simulink model "EV_ControlSystem_Architecture"  (R2025b)
settings: Solver=FixedStepAuto  StartTime=0.0  StopTime=inf  RelTol=1e-3
settings Model: DataDictionary=systemParams.sldd  Creator=smuckati  LastModifiedBy=smuckati
settings OptimizationCC: UseDivisionForNetSlopeComputation=on
settings DebuggingCC: ParameterPrecisionLossMsg=none
settings ModelReferenceCC: ModelReferenceNumInstancesAllowed=Single
settings RTWCC: GPUComputeCapability=3.5
settings GRTTargetCC: SubcomponentCodeInterfacePackaging=Nonreusable function

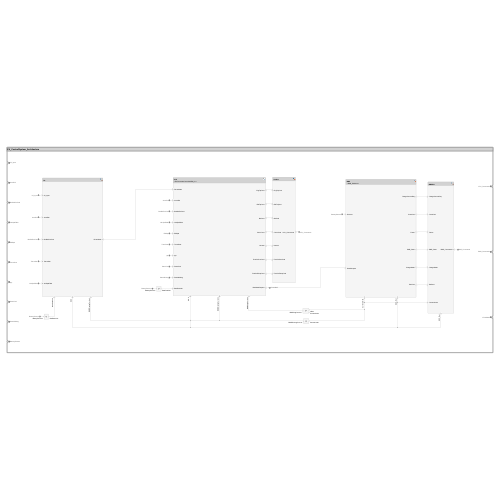
[thumbnail: Simulink's stored preview of the top-level diagram]
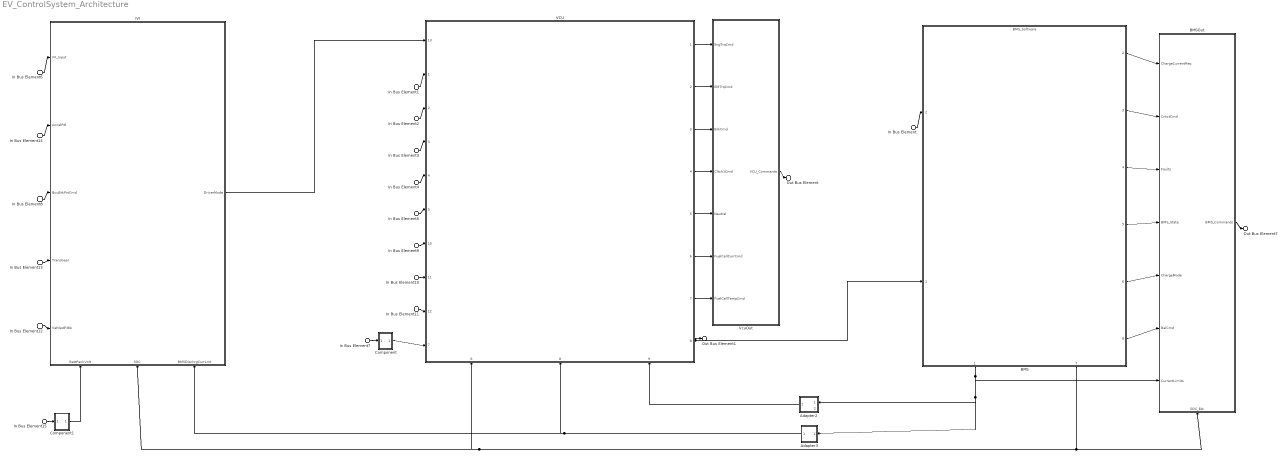
== system EV_ControlSystem_Architecture ==
  In Bus Element6 : Inport  PortName=IVI_Input
  In Bus Element1 : Inport  Port=2  PortName=AccelPdl
  In Bus Element14 : Inport  Port=2  PortName=AccelPdl
  In Bus Element2 : Inport  Port=3  PortName=BcuBrkPrsCmd
  In Bus Element8 : Inport  Port=3  PortName=BcuBrkPrsCmd
  In Bus Element3 : Inport  Port=4  PortName=VehSpdFdbk
  In Bus Element12 : Inport  Port=4  PortName=VehSpdFdbk
  In Bus Element4 : Inport  Port=5  PortName=EMSpd
  In Bus Element5 : Inport  Port=6  PortName=TransGear
  In Bus Element13 : Inport  Port=6  PortName=TransGear
  In Bus Element9 : Inport  Port=7  PortName=pqr
  In Bus Element10 : Inport  Port=8  PortName=SteerCmd
  In Bus Element11 : Inport  Port=9  PortName=SteerWhlAng
  In Bus Element : Inport  Port=10  PortName=BatterySensors
  In Bus Element7 : Inport  Port=10  PortName=BatterySensors
  In Bus Element15 : Inport  Port=10  PortName=BatterySensors
  Adapter2 : Subsystem
      settings: PortSchema="{\"entries\":[{\"content\":{\"margin\":10,\"minimumSpacing\":15,\"sides\":[{\"content\":{\"connectorIds\":[\"Out1\"]},\"type\":\"ConnectorPlacement.EquallySpacedRectSide\",\"uuid\":\"0bbc9e3d-7235-47d6-ad6f-dd1f8eb5ef8f\"},{\"content\":{\"connectorIds\":[\"In1\",\"In2\"],\"side\":\"RIGHT\"},\"type\":\"ConnectorPlacement.EquallySpacedRectSide\",\"uuid\":\"65cf6885-6ff6-4737-9f0f-48431dc9ec05\"},{\"content\":{\"side\":\"TOP\"},\"type\":\"ConnectorPlacement.EquallySpacedRectSide\",\"uuid\":\"345e4547-f67c-4bab-8588-ce41d45f9363\"}]},\"type\":\"ConnectorPlacement.EquallySpacedConnector\",\"uuid\":\"b8001fcd-770d-4504-9144-d19717d53d24\"}],\"packageUris\":[\"http://schema.mathworks.com/mf0/Connector/R2020b\"],\"version\":\"1.0\"}"
  Adapter3 : Subsystem
      settings: PortSchema="{\"entries\":[{\"content\":{\"margin\":10,\"minimumSpacing\":15,\"sides\":[{\"content\":{\"connectorIds\":[\"Out1\"]},\"type\":\"ConnectorPlacement.EquallySpacedRectSide\",\"uuid\":\"0bbc9e3d-7235-47d6-ad6f-dd1f8eb5ef8f\"},{\"content\":{\"connectorIds\":[\"In1\"],\"side\":\"RIGHT\"},\"type\":\"ConnectorPlacement.EquallySpacedRectSide\",\"uuid\":\"65cf6885-6ff6-4737-9f0f-48431dc9ec05\"},{\"content\":{\"side\":\"TOP\"},\"type\":\"ConnectorPlacement.EquallySpacedRectSide\",\"uuid\":\"345e4547-f67c-4bab-8588-ce41d45f9363\"}]},\"type\":\"ConnectorPlacement.EquallySpacedConnector\",\"uuid\":\"b8001fcd-770d-4504-9144-d19717d53d24\"}],\"packageUris\":[\"http://schema.mathworks.com/mf0/Connector/R2020b\"],\"version\":\"1.0\"}"
  BMS : ModelReference  ModelNameDialog=BMS_Software  SimulationMode=Normal  ModelReferenceVersion=11.4
      settings: PortSchema="{\"entries\":[{\"content\":{\"headerSize\":38,\"margin\":15,\"minimumSpacing\":25,\"sides\":[{\"content\":{\"connectorIds\":[\"In2\",\"In1\"]},\"type\":\"ConnectorPlacement.EquallySpacedRectSide\",\"uuid\":\"1684aa06-7c09-45e9-a207-933b45b16ad6\"},{\"content\":{\"connectorIds\":[\"Out2\",\"Out3\",\"Out4\",\"Out5\",\"Out6\",\"Out8\"],\"side\":\"RIGHT\"},\"type\":\"ConnectorPlacement.EquallySpacedRectSide\",\"uuid\":\"92a40eb6-ce6d-4197-95e5-619e5cbf745b\"},{\"content\":{\"side\":\"TOP\"},\"type\":\"ConnectorPlacement.EquallySpacedRectSide\",\"uuid\":\"e9ffeedd-dc68-477a-803d-14826416b02e\"},{\"content\":{\"connectorIds\":[\"Out1\",\"Out7\"],\"side\":\"BOTTOM\"},\"type\":\"ConnectorPlacement.EquallySpacedRectSide\",\"uuid\":\"a73cbf5d-dd2f-4f3b-b4a2-8c33c0d9382e\"}]},\"type\":\"ConnectorPlacement.EquallySpacedConnector\",\"uuid\":\"1901e345-f71e-4164-ad80-cf1092e39a7b\"}],\"packageUris\":[\"http://schema.mathworks.com/mf0/Connector/R2020b\"],\"version\":\"1.0\"}"
  BMSOut : Subsystem
      settings: PortSchema="{\"entries\":[{\"content\":{\"headerSize\":26,\"margin\":15,\"minimumSpacing\":25,\"sides\":[{\"content\":{\"connectorIds\":[\"In2\",\"In3\",\"In4\",\"In5\",\"In6\",\"In7\",\"In8\"]},\"type\":\"ConnectorPlacement.EquallySpacedRectSide\",\"uuid\":\"58a5bcb5-b5b6-43c9-9ab9-ad7b56807429\"},{\"content\":{\"connectorIds\":[\"Out1\"],\"side\":\"RIGHT\"},\"type\":\"ConnectorPlacement.EquallySpacedRectSide\",\"uuid\":\"182e3572-20a9-4903-88bd-08ae5ae4a66b\"},{\"content\":{\"side\":\"TOP\"},\"type\":\"ConnectorPlacement.EquallySpacedRectSide\",\"uuid\":\"b57b91fb-4a21-4ebf-b0d2-47c47f92b1a1\"},{\"content\":{\"connectorIds\":[\"In1\"],\"side\":\"BOTTOM\"},\"type\":\"ConnectorPlacement.EquallySpacedRectSide\",\"uuid\":\"ffc923e8-341b-44c7-96b0-eae8ed13ab76\"}]},\"type\":\"ConnectorPlacement.EquallySpacedConnector\",\"uuid\":\"fd34c378-6982-409c-b390-5cad93b9488e\"}],\"packageUris\":[\"http://schema.mathworks.com/mf0/Connector/R2020b\"],\"version\":\"1.0\"}"
  Component : Subsystem
      settings: PortSchema="{\"entries\":[{\"content\":{\"margin\":10,\"minimumSpacing\":15,\"sides\":[{\"content\":{\"connectorIds\":[\"In1\"]},\"type\":\"ConnectorPlacement.EquallySpacedRectSide\",\"uuid\":\"0bbc9e3d-7235-47d6-ad6f-dd1f8eb5ef8f\"},{\"content\":{\"connectorIds\":[\"Out1\"],\"side\":\"RIGHT\"},\"type\":\"ConnectorPlacement.EquallySpacedRectSide\",\"uuid\":\"65cf6885-6ff6-4737-9f0f-48431dc9ec05\"},{\"content\":{\"side\":\"TOP\"},\"type\":\"ConnectorPlacement.EquallySpacedRectSide\",\"uuid\":\"345e4547-f67c-4bab-8588-ce41d45f9363\"}]},\"type\":\"ConnectorPlacement.EquallySpacedConnector\",\"uuid\":\"b8001fcd-770d-4504-9144-d19717d53d24\"}],\"packageUris\":[\"http://schema.mathworks.com/mf0/Connector/R2020b\"],\"version\":\"1.0\"}"
  Component1 : Subsystem
      settings: PortSchema="{\"entries\":[{\"content\":{\"margin\":10,\"minimumSpacing\":15,\"sides\":[{\"content\":{\"connectorIds\":[\"In1\"]},\"type\":\"ConnectorPlacement.EquallySpacedRectSide\",\"uuid\":\"0bbc9e3d-7235-47d6-ad6f-dd1f8eb5ef8f\"},{\"content\":{\"connectorIds\":[\"Out1\"],\"side\":\"RIGHT\"},\"type\":\"ConnectorPlacement.EquallySpacedRectSide\",\"uuid\":\"65cf6885-6ff6-4737-9f0f-48431dc9ec05\"},{\"content\":{\"side\":\"TOP\"},\"type\":\"ConnectorPlacement.EquallySpacedRectSide\",\"uuid\":\"345e4547-f67c-4bab-8588-ce41d45f9363\"}]},\"type\":\"ConnectorPlacement.EquallySpacedConnector\",\"uuid\":\"b8001fcd-770d-4504-9144-d19717d53d24\"}],\"packageUris\":[\"http://schema.mathworks.com/mf0/Connector/R2020b\"],\"version\":\"1.0\"}"
  IVI : Subsystem
      settings: PortSchema="{\"entries\":[{\"content\":{\"headerSize\":26,\"margin\":15,\"minimumSpacing\":25,\"sides\":[{\"content\":{\"connectorIds\":[\"In1\",\"In4\",\"In8\",\"In6\",\"In5\"]},\"type\":\"ConnectorPlacement.EquallySpacedRectSide\",\"uuid\":\"1684aa06-7c09-45e9-a207-933b45b16ad6\"},{\"content\":{\"connectorIds\":[\"Out1\"],\"side\":\"RIGHT\"},\"type\":\"ConnectorPlacement.EquallySpacedRectSide\",\"uuid\":\"92a40eb6-ce6d-4197-95e5-619e5cbf745b\"},{\"content\":{\"side\":\"TOP\"},\"type\":\"ConnectorPlacement.EquallySpacedRectSide\",\"uuid\":\"e9ffeedd-dc68-477a-803d-14826416b02e\"},{\"content\":{\"connectorIds\":[\"In7\",\"In2\",\"In3\"],\"side\":\"BOTTOM\"},\"type\":\"ConnectorPlacement.EquallySpacedRectSide\",\"uuid\":\"a6cfa6b2-1e85-47f7-bf17-58c4213f5bb2\"}]},\"type\":\"ConnectorPlacement.EquallySpacedConnector\",\"uuid\":\"1901e345-f71e-4164-ad80-cf1092e39a7b\"}],\"packageUris\":[\"http://schema.mathworks.com/mf0/Connector/R2020b\"],\"version\":\"1.0\"}"
  VCU : Subsystem  ReferencedSubsystem=EvPowertrainController2EM_r3
      settings: PortSchema="{\"entries\":[{\"content\":{\"headerSize\":26,\"margin\":15,\"minimumSpacing\":25,\"sides\":[{\"content\":{\"connectorIds\":[\"In13\",\"In1\",\"In2\",\"In3\",\"In4\",\"In5\",\"In10\",\"In11\",\"In12\",\"In7\"]},\"type\":\"ConnectorPlacement.EquallySpacedRectSide\",\"uuid\":\"1684aa06-7c09-45e9-a207-933b45b16ad6\"},{\"content\":{\"connectorIds\":[\"Out1\",\"Out2\",\"Out3\",\"Out4\",\"Out5\",\"Out6\",\"Out7\",\"Out8\"],\"side\":\"RIGHT\"},\"type\":\"ConnectorPlacement.EquallySpacedRectSide\",\"uuid\":\"92a40eb6-ce6d-4197-95e5-619e5cbf745b\"},{\"content\":{\"side\":\"TOP\"},\"type\":\"ConnectorPlacement.EquallySpacedRectSide\",\"uuid\":\"e9ffeedd-dc68-477a-803d-14826416b02e\"},{\"content\":{\"connectorIds\":[\"In6\",\"In8\",\"In9\"],\"side\":\"BOTTOM\"},\"type\":\"ConnectorPlacement.EquallySpacedRectSide\",\"uuid\":\"0bc334ff-3cc8-4f87-96c9-e8251c73f7a2\"}]},\"type\":\"ConnectorPlacement.EquallySpacedConnector\",\"uuid\":\"1901e345-f71e-4164-ad80-cf1092e39a7b\"}],\"packageUris\":[\"http://schema.mathworks.com/mf0/Connector/R2020b\"],\"version\":\"1.0\"}"
  VcuOut : Subsystem
      settings: PortSchema="{\"entries\":[{\"content\":{\"headerSize\":26,\"margin\":15,\"minimumSpacing\":25,\"sides\":[{\"content\":{\"connectorIds\":[\"In1\",\"In2\",\"In3\",\"In4\",\"In5\",\"In6\",\"In7\"]},\"type\":\"ConnectorPlacement.EquallySpacedRectSide\",\"uuid\":\"58a5bcb5-b5b6-43c9-9ab9-ad7b56807429\"},{\"content\":{\"connectorIds\":[\"Out1\"],\"side\":\"RIGHT\"},\"type\":\"ConnectorPlacement.EquallySpacedRectSide\",\"uuid\":\"182e3572-20a9-4903-88bd-08ae5ae4a66b\"},{\"content\":{\"side\":\"TOP\"},\"type\":\"ConnectorPlacement.EquallySpacedRectSide\",\"uuid\":\"b57b91fb-4a21-4ebf-b0d2-47c47f92b1a1\"}]},\"type\":\"ConnectorPlacement.EquallySpacedConnector\",\"uuid\":\"fd34c378-6982-409c-b390-5cad93b9488e\"}],\"packageUris\":[\"http://schema.mathworks.com/mf0/Connector/R2020b\"],\"version\":\"1.0\"}"
  Out Bus Element : Outport  PortName=VCU_Commands
  Out Bus Element7 : Outport  Port=2  PortName=BMS_Commands
  Out Bus Element1 : Outport  Port=3  PortName=VCUtoBMS
  wires:
  In Bus Element/1 -> BMS/2
  VCU/8 -> Out Bus Element1/1, BMS/1
  BMS/7 -> VCU/6, IVI/2(SOC), BMSOut/1(SOC_Est)
  IVI/1(DriverMode) -> VCU/13
  BMS/1 -> Adapter3/1(CurrentLimits), Adapter2/1(InBus), BMSOut/8(CurrentLimits)
  In Bus Element1/1 -> VCU/1
  In Bus Element2/1 -> VCU/2
  In Bus Element3/1 -> VCU/3
  In Bus Element4/1 -> VCU/4
  In Bus Element5/1 -> VCU/5
  In Bus Element9/1 -> VCU/10
  In Bus Element10/1 -> VCU/11
  In Bus Element11/1 -> VCU/12
  Adapter2/1(BMSChrgCurrLmt) -> VCU/9
  Adapter3/1(BMSDischrgCurrLmt) -> VCU/8, IVI/3(BMSDischrgCurrLmt)
  In Bus Element7/1 -> Component/1(BatterySensors)
  Component/1(BattPackVolt) -> VCU/7
  In Bus Element6/1 -> IVI/1(IVI_Input)
  In Bus Element8/1 -> IVI/8(BcuBrkPrsCmd)
  In Bus Element12/1 -> IVI/5(VehSpdFdbk)
  In Bus Element13/1 -> IVI/6(TransGear)
  In Bus Element14/1 -> IVI/4(AccelPdl)
  In Bus Element15/1 -> Component1/1(BatterySensors)
  Component1/1(BattPackVolt) -> IVI/7(BattPackVolt)
  VCU/3 -> VcuOut/3(BrkCmd)
  VCU/4 -> VcuOut/4(Cltch1Cmd)
  VCU/2 -> VcuOut/2(EMTrqCmd)
  VCU/1 -> VcuOut/1(EngTrqCmd)
  VCU/6 -> VcuOut/6(FuelCellCurrCmd)
  VCU/7 -> VcuOut/7(FuelCellTempCmd)
  VCU/5 -> VcuOut/5(Neutral)
  VcuOut/1(VCU_Commands) -> Out Bus Element/1
  BMS/5 -> BMSOut/5(BMS_State)
  BMS/8 -> BMSOut/7(BalCmd)
  BMS/2 -> BMSOut/2(ChargeCurrentReq)
  BMS/6 -> BMSOut/6(ChargeMode)
  BMS/3 -> BMSOut/3(CntctCmd)
  BMS/4 -> BMSOut/4(Faults)
  BMSOut/1(BMS_Commands) -> Out Bus Element7/1

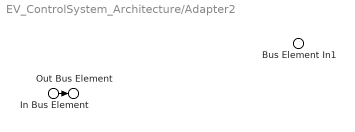
== system EV_ControlSystem_Architecture/Adapter2 ==
  Bus Element In1 : Inport  PortName=InBus
  In Bus Element : Inport  Port=2  PortName=CurrentLimits  Element=ChargeCurrentLimit
  Out Bus Element : Outport  PortName=BMSChrgCurrLmt  Element=ChargeCurrentLimit
  wires:
  In Bus Element/1 -> Out Bus Element/1

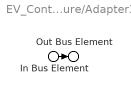
== system EV_ControlSystem_Architecture/Adapter3 ==
  In Bus Element : Inport  PortName=CurrentLimits  Element=DischargeCurrentLimit
  Out Bus Element : Outport  PortName=BMSDischrgCurrLmt  Element=DischargeCurrentLimit
  wires:
  In Bus Element/1 -> Out Bus Element/1

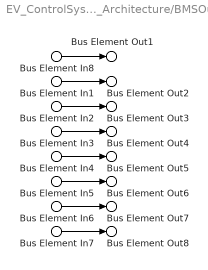
== system EV_ControlSystem_Architecture/BMSOut ==
  Bus Element In8 : Inport  PortName=SOC_Est
  Bus Element In1 : Inport  Port=2  PortName=ChargeCurrentReq
  Bus Element In2 : Inport  Port=3  PortName=CntctCmd
  Bus Element In3 : Inport  Port=4  PortName=Faults
  Bus Element In4 : Inport  Port=5  PortName=BMS_State
  Bus Element In5 : Inport  Port=6  PortName=ChargeMode
  Bus Element In6 : Inport  Port=7  PortName=BalCmd
  Bus Element In7 : Inport  Port=8  PortName=CurrentLimits
  Bus Element Out1 : Outport  PortName=BMS_Commands  Element=SOC
  Bus Element Out2 : Outport  PortName=BMS_Commands  Element=ChargeCurrentReq
  Bus Element Out3 : Outport  PortName=BMS_Commands  Element=CntctCmd
  Bus Element Out4 : Outport  PortName=BMS_Commands  Element=Faults
  Bus Element Out5 : Outport  PortName=BMS_Commands  Element=BMS_State
  Bus Element Out6 : Outport  PortName=BMS_Commands  Element=ChargeMode
  Bus Element Out7 : Outport  PortName=BMS_Commands  Element=BalCmd
  Bus Element Out8 : Outport  PortName=BMS_Commands  Element=CurrentLimits
  wires:
  Bus Element In8/1 -> Bus Element Out1/1
  Bus Element In1/1 -> Bus Element Out2/1
  Bus Element In2/1 -> Bus Element Out3/1
  Bus Element In3/1 -> Bus Element Out4/1
  Bus Element In4/1 -> Bus Element Out5/1
  Bus Element In5/1 -> Bus Element Out6/1
  Bus Element In6/1 -> Bus Element Out7/1
  Bus Element In7/1 -> Bus Element Out8/1

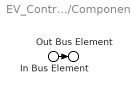
== system EV_ControlSystem_Architecture/Component ==
  In Bus Element : Inport  PortName=BatterySensors  Element=Pack_Voltage
  Out Bus Element : Outport  PortName=BattPackVolt  Element=Pack_Voltage
  wires:
  In Bus Element/1 -> Out Bus Element/1

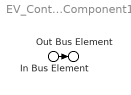
== system EV_ControlSystem_Architecture/Component1 ==
  In Bus Element : Inport  PortName=BatterySensors  Element=Pack_Voltage
  Out Bus Element : Outport  PortName=BattPackVolt  Element=Pack_Voltage
  wires:
  In Bus Element/1 -> Out Bus Element/1

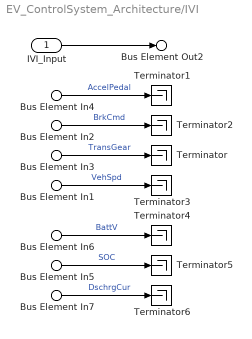
== system EV_ControlSystem_Architecture/IVI ==
  IVI_Input : Inport  OutDataTypeStr=Enum: DriverMode
  Bus Element In5 : Inport  Port=2  PortName=SOC
  Bus Element In7 : Inport  Port=3  PortName=BMSDischrgCurrLmt
  Bus Element In4 : Inport  Port=4  PortName=AccelPdl
  Bus Element In1 : Inport  Port=5  PortName=VehSpdFdbk
  Bus Element In3 : Inport  Port=6  PortName=TransGear
  Bus Element In6 : Inport  Port=7  PortName=BattPackVolt
  Bus Element In2 : Inport  Port=8  PortName=BcuBrkPrsCmd
  Terminator{,1..6} (7 alike) : Terminator
  Bus Element Out2 : Outport  PortName=DriverMode
  wires:
  IVI_Input/1 -> Bus Element Out2/1
  Bus Element In3/1 -> Terminator/1  "TransGear"
  Bus Element In4/1 -> Terminator1/1  "AccelPedal"
  Bus Element In2/1 -> Terminator2/1  "BrkCmd"
  Bus Element In1/1 -> Terminator3/1  "VehSpd"
  Bus Element In6/1 -> Terminator4/1  "BattV"
  Bus Element In5/1 -> Terminator5/1  "SOC"
  Bus Element In7/1 -> Terminator6/1  "DschrgCur"

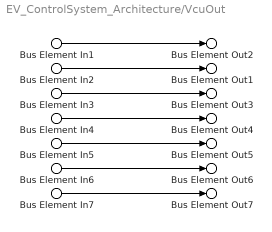
== system EV_ControlSystem_Architecture/VcuOut ==
  Bus Element In1 : Inport  PortName=EngTrqCmd
  Bus Element In2 : Inport  Port=2  PortName=EMTrqCmd
  Bus Element In3 : Inport  Port=3  PortName=BrkCmd
  Bus Element In4 : Inport  Port=4  PortName=Cltch1Cmd
  Bus Element In5 : Inport  Port=5  PortName=Neutral
  Bus Element In6 : Inport  Port=6  PortName=FuelCellCurrCmd
  Bus Element In7 : Inport  Port=7  PortName=FuelCellTempCmd
  Bus Element Out2 : Outport  PortName=VCU_Commands  Element=EngTrqCmd
  Bus Element Out1 : Outport  PortName=VCU_Commands  Element=EMTrqCmd
  Bus Element Out3 : Outport  PortName=VCU_Commands  Element=BrkCmd
  Bus Element Out4 : Outport  PortName=VCU_Commands  Element=Cltch1Cmd
  Bus Element Out5 : Outport  PortName=VCU_Commands  Element=Neutral
  Bus Element Out6 : Outport  PortName=VCU_Commands  Element=FuelCellCurrCmd
  Bus Element Out7 : Outport  PortName=VCU_Commands  Element=FuelCellTempCmd
  wires:
  Bus Element In7/1 -> Bus Element Out7/1
  Bus Element In1/1 -> Bus Element Out2/1
  Bus Element In2/1 -> Bus Element Out1/1
  Bus Element In3/1 -> Bus Element Out3/1
  Bus Element In4/1 -> Bus Element Out4/1
  Bus Element In5/1 -> Bus Element Out5/1
  Bus Element In6/1 -> Bus Element Out6/1
